simulink model "model8Kratadobre"  (Simulink 6.6)
settings: Solver=ode45  StartTime=0.0  StopTime=250  MaxStep=0.01  MinStep=0.001  RelTol=1e-6
values from neighbouring files (symbols this model uses):
  a1 = w1/w0    (= 84)    [dane8Krata.m]
  a2 = w2/w0    (= 273)    [dane8Krata.m]
  a3 = 1/w0    (= 180)    [dane8Krata.m]
  b0 = d12*d23 / (C1*w0)    (= 3)    [dane8Krata.m]
  kp1 = 0.5*kg    (= 21.05)    [dane8Krata.m]
  kp2 = 0.45*kg    (= 18.945)    [dane8Krata.m]
  kp3 = 0.6*kg    (= 25.26)    [dane8Krata.m]
  p0 = 1    [dane8Krata.m]
  Td3 = Tg/8    (= 1.15875)    [dane8Krata.m]
  Ti2 = Tg/1.2    (= 7.725)    [dane8Krata.m]
  Ti3 = Tg/2    (= 4.635)    [dane8Krata.m]
libraries: simulink_extras x3
settings Model: Creator=Administrator  LastModifiedBy=Damian
settings DataIOCC: LimitDataPoints=off
settings DebuggingCC: SignalResolutionControl=TryResolveAllWithWarning  MultiTaskDSMMsg=warning  MultiTaskCondExecSysMsg=none  StrictBusMsg=None
settings RTWCC: IncludeERTFirstTime=on

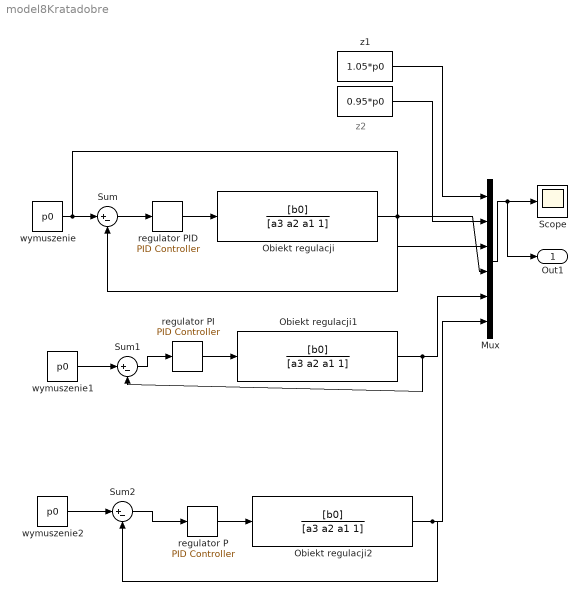
== system model8Kratadobre ==
  note: z2
  " " : Constant  Value=0.95*p0
  Mux : Mux  Inputs=6
  Obiekt regulacji : TransferFcn  Numerator=[b0]  Denominator=[a3 a2 a1 1]
  Obiekt regulacji1 : TransferFcn  Numerator=[b0]  Denominator=[a3 a2 a1 1]
  Obiekt regulacji2 : TransferFcn  Numerator=[b0]  Denominator=[a3 a2 a1 1]
  Scope : Scope
      settings: YMin=-100000  YMax=100000
  Sum : Sum  Inputs=|+-
  Sum1 : Sum  Inputs=|+-
  Sum2 : Sum  Inputs=|+-
  regulator P : simulink_extras/Additional Linear/PID Controller  SystemSampleTime=-1  P=kp1  I=0  D=0
  regulator PI : simulink_extras/Additional Linear/PID Controller  SystemSampleTime=-1  P=kp2  I=kp2/Ti2  D=0
  regulator PID : simulink_extras/Additional Linear/PID Controller  SystemSampleTime=-1  P=kp3  I=kp3/Ti3  D=Td3*kp3
  wymuszenie : Constant  Value=p0
  wymuszenie1 : Constant  Value=p0
  wymuszenie2 : Constant  Value=p0
  z1 : Constant  Value=1.05*p0
  Out1 : Outport
  wires:
  wymuszenie/1 -> Sum/1, Mux/3
  Mux/1 -> Scope/1, Out1/1
  Sum/1 -> regulator PID/1
  regulator PID/1 -> Obiekt regulacji/1
  Obiekt regulacji/1 -> Sum/2, Mux/4
  " "/1 -> Mux/2
  z1/1 -> Mux/1
  regulator PI/1 -> Obiekt regulacji1/1
  regulator P/1 -> Obiekt regulacji2/1
  Obiekt regulacji1/1 -> Mux/5, Sum1/2
  Obiekt regulacji2/1 -> Mux/6, Sum2/2
  wymuszenie1/1 -> Sum1/1
  wymuszenie2/1 -> Sum2/1
  Sum1/1 -> regulator PI/1
  Sum2/1 -> regulator P/1
